simulink model "carModel"  (R2021a)
settings: Solver=ode15s  StartTime=0.0  StopTime=50  MaxStep=0.5  RelTol=1e-3
values from neighbouring files (symbols this model uses):
  initialFuel = 100    [data.m]
  maxEngineTemp = 240    [data.m]
  maxEngineTorque = 80    [data.m]
  maxMotorTemp = 135    [data.m]
  maxMotorTorque = 80    [data.m]
  maxRegenTorque = 80    [data.m]
  motorVoltage = 140    [data.m]
undefined symbols (not defined in the file or in its folder): b, k, Lock, N, sigbuilder_block, Temp_bpts, up
libraries: autolibsharedcoupling x7, autolibshared x7, autolibpowerinfoutils x4, autolibshareddiff x3, autolibhevctrlrcommon x2, autolibtrqconv x2, autolibutils x2, autolibtransamt x1, autolibsharedtransfixedgear x1, autolibdcdc x1, autolibdatasheetbattery x1, autolibmappedmotor x1
(part 6 of 6)

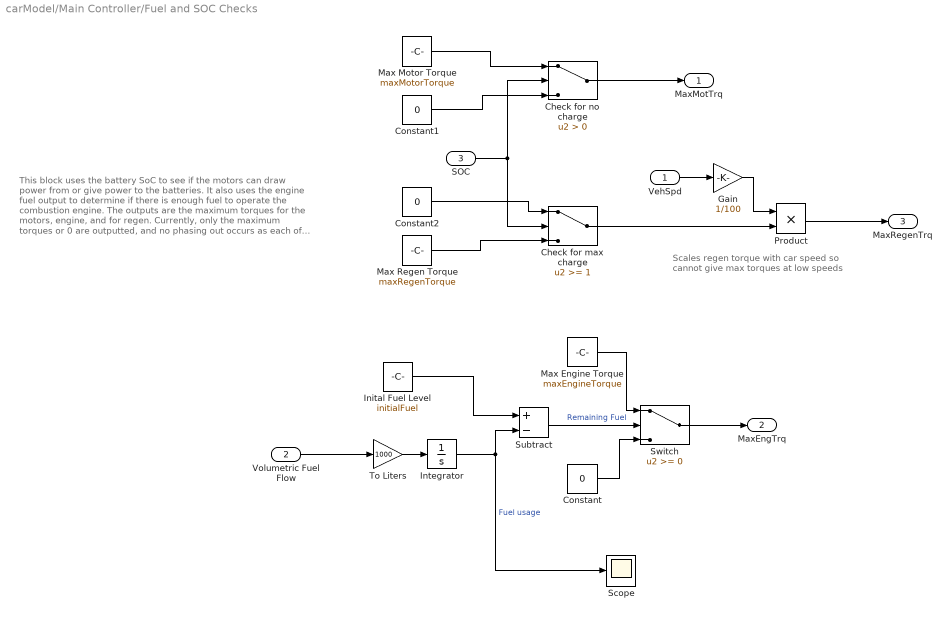
== system carModel/Main Controller/Fuel and SOC Checks ==
  note: Scales regen torque with car speed
      | so cannot give max torques at low speeds
  note: This block uses the battery SoC to see if the motors can draw power from or give power to the batteries. It also uses the engine fuel output to determine if there is enough fuel to operate the combustion engine. The outputs are the maximum torques for the motors, engine, and for regen.
      |
      | Currently, only the maximum torques or 0 are outputted, and no phasing out occurs as each of the power supply decreases.
  VehSpd : Inport
  Volumetric Fuel Flow : Inport  Port=2
  SOC : Inport  Port=3
  Check for max charge : Switch  Threshold=1
  Check for no charge : Switch  Criteria=u2 > Threshold
  Constant : Constant  Value=0
  Constant1 : Constant  Value=0
  Constant2 : Constant  Value=0
  Gain : Gain  Gain=1/100
  Inital Fuel Level : Constant  Value=initialFuel
  Integrator : Integrator
  Max Engine Torque : Constant  Value=maxEngineTorque
  Max Motor Torque : Constant  Value=maxMotorTorque
  Max Regen Torque : Constant  Value=maxRegenTorque
  Product : Product
  Scope : Scope
  Subtract : Sum  Inputs=+-
  Switch : Switch
  To Liters : Gain  Gain=1000
  MaxMotTrq : Outport
  MaxEngTrq : Outport  Port=2
  MaxRegenTrq : Outport  Port=3
  wires:
  Subtract/1 -> Switch/2  "Remaining Fuel"
  Constant/1 -> Switch/3
  Inital Fuel Level/1 -> Subtract/1
  Integrator/1 -> Scope/1, Subtract/2  "Fuel usage"
  Volumetric Fuel Flow/1 -> To Liters/1
  Max Engine Torque/1 -> Switch/1
  Switch/1 -> MaxEngTrq/1
  Check for no charge/1 -> MaxMotTrq/1
  Max Motor Torque/1 -> Check for no charge/1
  Constant1/1 -> Check for no charge/3
  SOC/1 -> Check for max charge/2, Check for no charge/2
  Max Regen Torque/1 -> Check for max charge/3
  Constant2/1 -> Check for max charge/1
  Check for max charge/1 -> Product/2
  VehSpd/1 -> Gain/1
  Product/1 -> MaxRegenTrq/1
  Gain/1 -> Product/1
  To Liters/1 -> Integrator/1

== system carModel/Main Controller/Heat Controller ==
  note: Decreases the torque to the motor or engine if they are overheating by the power of the stand-in gain function.
      | This system doesn't make the other motor/engine work harder if one is too hot. Therefore when one is overheated the car instantly loses power, instead of when both are overheated.
  Motor Torque : Inport
  Engine Torque : Inport  Port=2
  Engine Temp Switch : Switch  Criteria=u2 > Threshold  Threshold=maxEngineTemp
  Motor Temp Switch : Switch  Criteria=u2 > Threshold  Threshold=maxMotorTemp
  Signal Builder : Subsystem  Tag=STV Subsys  LoadFcn=sigbuilder_block('load');  StartFcn=sigbuilder_block('start');  StopFcn=sigbuilder_block('stop');  ClipboardFcn=sigbuilder_block('clipboard');  mask(Sigbuilder block){tuvar=[0:10]}
      mask help: Simulink:masks:SigbuilderBlock_MD
      mask init:
      | if ~strcmp(get_param(bdroot(gcbh),'SimulationStatus'),'stopped') tuvar = sigbuilder_block('maskInit'); end
      settings: CopyFcn=sigbuilder_block('copy');  DeleteFcn=sigbuilder_block('delete');  ModelCloseFcn=sigbuilder_block('modelClose');  PreSaveFcn=sigbuilder_block('preSave');  PauseFcn=sigbuilder_block('pause');  ContinueFcn=sigbuilder_block('continue');  NameChangeFcn=sigbuilder_block('namechange');  OpenFcn=sigbuilder_block('open',[411 128.5 543.5 351.5 ]);  CloseFcn=sigbuilder_block('close');
      mask Display: plot(0, 0, 100, 100,[2, 2, 32, 32, 2], [68, 8, 8, 68, 68],[32, 2], [38, 38], [32, 19, 2],[53, 60, 44], [32, 17, 17, 2],[16, 16, 31, 31]);txt = getActiveGroup(gcbh);text(2, 100, txt,'verticalAlignment', 'top');
  place-holder to decrease engine torque : Gain
  place-holder to decrease motor torque : Gain
  Updated Motor Torque : Outport
  Updated Engine Torque : Outport  Port=2
  wires:
  Motor Torque/1 -> place-holder to decrease motor torque/1, Motor Temp Switch/3
  place-holder to decrease motor torque/1 -> Motor Temp Switch/1
  Engine Torque/1 -> place-holder to decrease engine torque/1, Engine Temp Switch/3
  place-holder to decrease engine torque/1 -> Engine Temp Switch/1
  Signal Builder/1(Motor temp) -> Motor Temp Switch/2
  Signal Builder/2(Engine temp) -> Engine Temp Switch/2
  Motor Temp Switch/1 -> Updated Motor Torque/1
  Engine Temp Switch/1 -> Updated Engine Torque/1

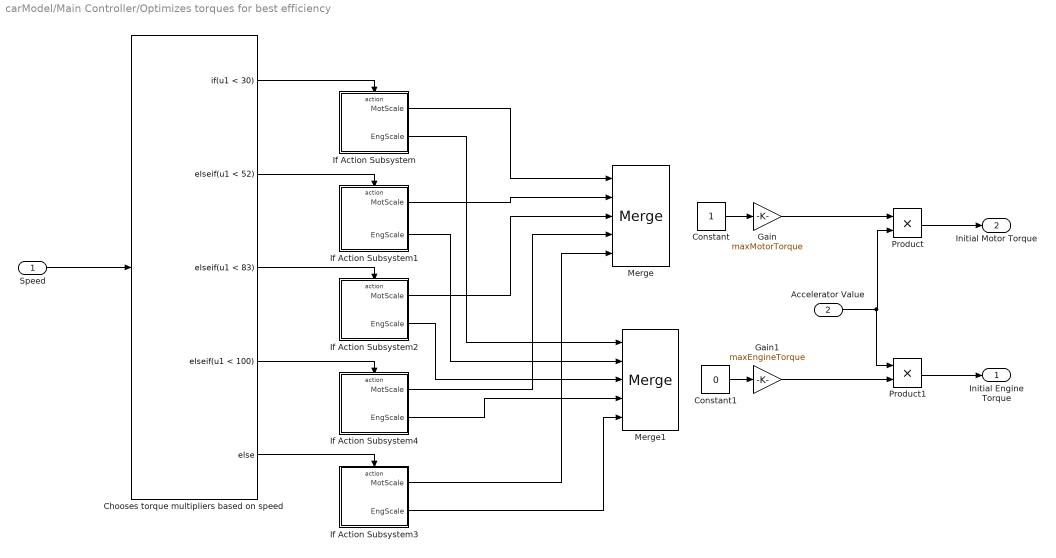
== system carModel/Main Controller/Optimizes torques for best efficiency ==
  Speed : Inport
  Accelerator Value : Inport  Port=2
  Chooses torque multipliers based on speed : If  IfExpression=u1 < 30  ElseIfExpressions=u1 < 52, u1 < 83, u1 < 100
  Constant : Constant
  Constant1 : Constant  Value=0
  Gain : Gain  Gain=maxMotorTorque
  Gain1 : Gain  Gain=maxEngineTorque
  If Action Subsystem : Subsystem  TreatAsAtomicUnit=on
  If Action Subsystem1 : Subsystem  TreatAsAtomicUnit=on
  If Action Subsystem2 : Subsystem  TreatAsAtomicUnit=on
  If Action Subsystem3 : Subsystem  TreatAsAtomicUnit=on
  If Action Subsystem4 : Subsystem  TreatAsAtomicUnit=on
  Merge : Merge  Inputs=5
  Merge1 : Merge  Inputs=5
  Product : Product
  Product1 : Product
  Initial Engine Torque : Outport
  Initial Motor Torque : Outport  Port=2
  wires:
  Speed/1 -> Chooses torque multipliers based on speed/1
  Accelerator Value/1 -> Product1/1, Product/2
  Product1/1 -> Initial Engine Torque/1
  Product/1 -> Initial Motor Torque/1
  Gain1/1 -> Product1/2
  Gain/1 -> Product/1
  Chooses torque multipliers based on speed/1 -> If Action Subsystem/Action
  Chooses torque multipliers based on speed/2 -> If Action Subsystem1/Action
  Chooses torque multipliers based on speed/3 -> If Action Subsystem2/Action
  Chooses torque multipliers based on speed/4 -> If Action Subsystem4/Action
  Chooses torque multipliers based on speed/5 -> If Action Subsystem3/Action
  If Action Subsystem/1(MotScale) -> Merge/1
  If Action Subsystem1/1(MotScale) -> Merge/2
  If Action Subsystem2/1(MotScale) -> Merge/3
  If Action Subsystem4/1(MotScale) -> Merge/4
  If Action Subsystem3/1(MotScale) -> Merge/5
  If Action Subsystem/2(EngScale) -> Merge1/1
  If Action Subsystem1/2(EngScale) -> Merge1/2
  If Action Subsystem2/2(EngScale) -> Merge1/3
  If Action Subsystem4/2(EngScale) -> Merge1/4
  If Action Subsystem3/2(EngScale) -> Merge1/5
  Constant/1 -> Gain/1
  Constant1/1 -> Gain1/1

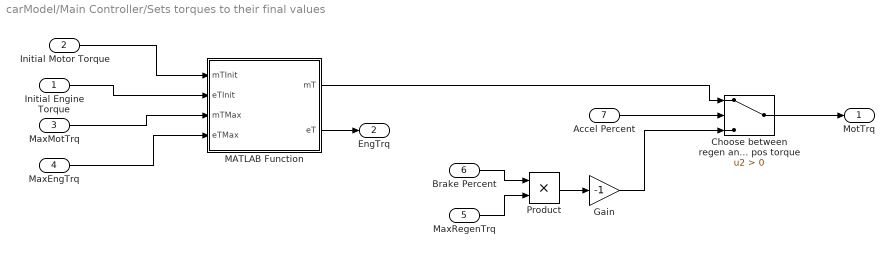
== system carModel/Main Controller/Sets torques to their final values ==
  Initial Engine Torque : Inport
  Initial Motor Torque : Inport  Port=2
  MaxMotTrq : Inport  Port=3
  MaxEngTrq : Inport  Port=4
  MaxRegenTrq : Inport  Port=5
  Brake Percent : Inport  Port=6
  Accel Percent : Inport  Port=7
  Choose between regen and pos torque : Switch  Criteria=u2 > Threshold
  Gain : Gain  Gain=-1
  MATLAB Function : MATLAB Function  TreatAsAtomicUnit=on
  Product : Product
  MotTrq : Outport
  EngTrq : Outport  Port=2
  wires:
  Gain/1 -> Choose between regen and pos torque/3
  MaxMotTrq/1 -> MATLAB Function/3(mTMax)
  MaxEngTrq/1 -> MATLAB Function/4(eTMax)
  Product/1 -> Gain/1
  Choose between regen and pos torque/1 -> MotTrq/1
  Brake Percent/1 -> Product/1
  Accel Percent/1 -> Choose between regen and pos torque/2
  MaxRegenTrq/1 -> Product/2
  Initial Motor Torque/1 -> MATLAB Function/1(mTInit)
  Initial Engine Torque/1 -> MATLAB Function/2(eTInit)
  MATLAB Function/2(eT) -> EngTrq/1
  MATLAB Function/1(mT) -> Choose between regen and pos torque/1

== system carModel/SI Engine/Accessory Load Model ==
  EngTrqIn : Inport
  EngSpd : Inport  Port=2
  Accessory Load Model : autolibhevctrlrcommon/Accessory Load Model  AccPwrTbl=[0 0]  AccSpdBpts=[300 750]
      settings: SourceProductBaseCode=PW
  Lumped Torque Dynamics : TransferFcn  Denominator=[0.2 1]
  Net Torque : Sum  Inputs=+-
  EngTrqOut : Outport  Unit=N*m  VectorParamsAs1DForOutWhenUnconnected=off
  wires:
  EngSpd/1 -> Accessory Load Model/1
  Lumped Torque Dynamics/1 -> EngTrqOut/1
  Net Torque/1 -> Lumped Torque Dynamics/1
  EngTrqIn/1 -> Net Torque/1
  Accessory Load Model/1 -> Net Torque/2

== system carModel/Drivetrain/Differential/Rear Axle Compliance 2 ==
  Info : Inport
  Bus Selector1 : BusSelector  OutputSignals=Trq.R,Trq.C
  Terminator : Terminator
  Terminator1 : Terminator
  Two-Way Connection1 : TwoWayConnection
  Two-Way Connection4 : TwoWayConnection
  R : PMIOPort  Side=Left
  C : PMIOPort  Port=2  Side=Right
  wires:
  Bus Selector1/2 -> Two-Way Connection1/1  "<C>"
  Bus Selector1/1 -> Two-Way Connection4/1  "<R>"
  Two-Way Connection1/1 -> Terminator1/1
  Info/1 -> Bus Selector1/1
  Two-Way Connection4/1 -> Terminator/1
  connections:
  Two-Way Connection1/RConn1 -- C/RConn1
  R/RConn1 -- Two-Way Connection4/RConn1

== system carModel/Drivetrain/Differential and Compliance/Front Axle Compliance 2 ==
  Info : Inport
  Bus Selector : BusSelector  OutputSignals=PwrInfo.PwrTrnsfrd,PwrInfo.PwrNotTrnsfrd,PwrInfo.PwrStored
  Bus Selector1 : BusSelector  OutputSignals=Trq.R,Trq.C
  Power Accounting Bus Creator : autolibpowerinfoutils/Power Accounting Bus Creator  AssctBlkSelPopup=Parent  RefBlkName='libraryname/blkname'  PwrTrnsfrdCheckBox=on  PwrNotTrnsfrdCheckBox=on  PwrStoredCheckBox=on  aMode=aMode
      settings: SourceProductBaseCode=PW,DR,MT,UV,VE
  Terminator : Terminator
  Terminator1 : Terminator
  Terminator2 : Terminator
  Two-Way Connection1 : TwoWayConnection
  Two-Way Connection4 : TwoWayConnection
  R : PMIOPort  Side=Left
  C : PMIOPort  Port=2  Side=Right
  wires:
  Bus Selector/3 -> Power Accounting Bus Creator/3  "<PwrStored>"
  Bus Selector/2 -> Power Accounting Bus Creator/2  "<PwrNotTrnsfrd>"
  Bus Selector/1 -> Power Accounting Bus Creator/1  "<PwrTrnsfrd>"
  Power Accounting Bus Creator/1 -> Terminator2/1
  Bus Selector1/2 -> Two-Way Connection1/1  "<C>"
  Bus Selector1/1 -> Two-Way Connection4/1  "<R>"
  Two-Way Connection1/1 -> Terminator1/1
  Info/1 -> Bus Selector/1, Bus Selector1/1
  Two-Way Connection4/1 -> Terminator/1
  connections:
  Two-Way Connection1/RConn1 -- C/RConn1
  R/RConn1 -- Two-Way Connection4/RConn1

== system carModel/Drivetrain/Differential and Compliance/Rear Axle Compliance 2 ==
  Info : Inport
  Bus Selector : BusSelector  OutputSignals=PwrInfo.PwrTrnsfrd,PwrInfo.PwrNotTrnsfrd,PwrInfo.PwrStored
  Bus Selector1 : BusSelector  OutputSignals=Trq.R,Trq.C
  Power Accounting Bus Creator : autolibpowerinfoutils/Power Accounting Bus Creator  AssctBlkSelPopup=Parent  RefBlkName='libraryname/blkname'  PwrTrnsfrdCheckBox=on  PwrNotTrnsfrdCheckBox=on  PwrStoredCheckBox=on  aMode=aMode
      settings: SourceProductBaseCode=PW,DR,MT,UV,VE
  Terminator : Terminator
  Terminator1 : Terminator
  Terminator2 : Terminator
  Two-Way Connection1 : TwoWayConnection
  Two-Way Connection4 : TwoWayConnection
  R : PMIOPort  Side=Left
  C : PMIOPort  Port=2  Side=Right
  wires:
  Bus Selector/3 -> Power Accounting Bus Creator/3  "<PwrStored>"
  Bus Selector/2 -> Power Accounting Bus Creator/2  "<PwrNotTrnsfrd>"
  Bus Selector/1 -> Power Accounting Bus Creator/1  "<PwrTrnsfrd>"
  Power Accounting Bus Creator/1 -> Terminator2/1
  Bus Selector1/2 -> Two-Way Connection1/1  "<C>"
  Bus Selector1/1 -> Two-Way Connection4/1  "<R>"
  Two-Way Connection1/1 -> Terminator1/1
  Info/1 -> Bus Selector/1, Bus Selector1/1
  Two-Way Connection4/1 -> Terminator/1
  connections:
  Two-Way Connection1/RConn1 -- C/RConn1
  R/RConn1 -- Two-Way Connection4/RConn1

== system carModel/Drivetrain/Transmission/Accessory Load Model1 ==
  EngTrqIn : Inport
  EngSpd : Inport  Port=2
  Accessory Load Model : autolibhevctrlrcommon/Accessory Load Model  AccPwrTbl=[0 0]  AccSpdBpts=[300 750]
      settings: SourceProductBaseCode=PW
  Lumped Torque Dynamics : TransferFcn  Denominator=[0.2 1]
  Net Torque : Sum  Inputs=+-
  EngTrqOut : Outport  Unit=N*m  VectorParamsAs1DForOutWhenUnconnected=off
  wires:
  EngSpd/1 -> Accessory Load Model/1
  Lumped Torque Dynamics/1 -> EngTrqOut/1
  Net Torque/1 -> Lumped Torque Dynamics/1
  EngTrqIn/1 -> Net Torque/1
  Accessory Load Model/1 -> Net Torque/2

== system carModel/Drivetrain/Transmission/Subsystem ==
  note: Gear Selection based on current vehicle speed
  VehSpdFdbk : Inport
  Gear 0 : Subsystem  TreatAsAtomicUnit=on
  Gear 1 : Subsystem  TreatAsAtomicUnit=on
  Gear 2 : Subsystem  TreatAsAtomicUnit=on
  Gear 3 : Subsystem  TreatAsAtomicUnit=on
  Gear 4 : Subsystem  TreatAsAtomicUnit=on
  Gear 5 : Subsystem  TreatAsAtomicUnit=on
  Gear Chooser : If  IfExpression=u1 == 0  ElseIfExpressions=u1 < 49.31, u1 < 60.69, u1 < 73.70, u1 < 88.70
  Selected Gear Merger : Merge  Inputs=6
  Gear : Outport
  wires:
  VehSpdFdbk/1 -> Gear Chooser/1
  Selected Gear Merger/1 -> Gear/1
  Gear 1/1(Out1) -> Selected Gear Merger/2
  Gear 2/1(Out1) -> Selected Gear Merger/3
  Gear 3/1(Out1) -> Selected Gear Merger/4
  Gear 4/1(Out1) -> Selected Gear Merger/5
  Gear 5/1(Out1) -> Selected Gear Merger/6
  Gear Chooser/5 -> Gear 4/Action
  Gear Chooser/6 -> Gear 5/Action
  Gear Chooser/4 -> Gear 3/Action
  Gear Chooser/3 -> Gear 2/Action
  Gear Chooser/2 -> Gear 1/Action
  Gear Chooser/1 -> Gear 0/Action
  Gear 0/1(Out1) -> Selected Gear Merger/1

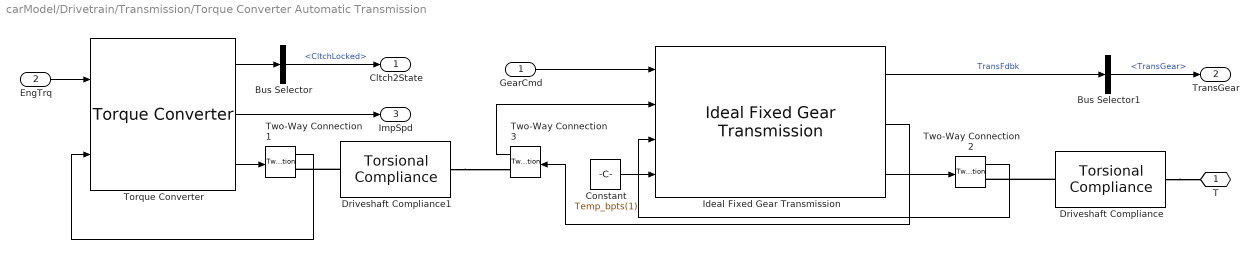
== system carModel/Drivetrain/Transmission/Torque Converter Automatic Transmission ==
  GearCmd : Inport
  EngTrq : Inport  Port=2
  Bus Selector : BusSelector  OutputSignals=Cltch.CltchLocked
  Bus Selector1 : BusSelector  OutputSignals=Trans.TransGear
  Constant : Constant  Value=Temp_bpts(1)
  Driveshaft Compliance : autolibsharedcoupling/Torsional Compliance  port_config=Two-way connection  extInfo=off  k=k  b=b  theta_o=theta_o  domega_o=domega_o  omega_c=omega_c  blkID=0  aMode=1
      settings: SourceProductBaseCode=PW,DR,MT,UV,VE
  Driveshaft Compliance1 : autolibsharedcoupling/Torsional Compliance  port_config=Two-way connection  extInfo=off  k=k  b=b  theta_o=theta_o  domega_o=domega_o  omega_c=omega_c  blkID=0  aMode=1
      settings: SourceProductBaseCode=PW,DR,MT,UV,VE
  Ideal Fixed Gear Transmission : autolibsharedtransfixedgear/Ideal Fixed Gear Transmission  VariantControl=0  TransEffModelPopup=Gear, input torque, input speed, and temperature  gearInterp=Linear point-slope  G=G  Trq_bpts=Trq_bpts  omega_bpts=omega_bpts  Temp_bpts=Temp_bpts  N=N  Jout=Jout  bout=bout  eta=eta  eta_tbl=eta_tbl  G_o=0  omega_o=omega_o  omegaN_o=0  tau_s=tau_s  maxAbsSpd=5e3  aMode=1
      settings: SourceProductBaseCode=PW,DR,MT,UV,VE
  Torque Converter : autolibtrqconv/Torque Converter  TCType=Lock-up  port_config=Simulink  Ji=Ji  bi=bi  Jt=Jt  bt=bt  omegai_o=omegai_o  omegat_o=omegat_o  phi=phi  KType=Input speed / sqrt(input torque)  psi=psi  zeta=zeta  tauTC=tauTC  InterpMethod=Linear  Reff=Reff  mus=mus  muk=muk  ClutchLocked=off  philu=philu  omegal=omegal  omegau=omegau  K_c=K_c  tauC=tauC  maxAbsSpd=5e3  tau_dl=3000
      settings: AttributesFormatString="Lock-up type:  %<TCType>"  SourceProductBaseCode=PW
  Two-Way Connection1 : TwoWayConnection
  Two-Way Connection2 : TwoWayConnection
  Two-Way Connection3 : TwoWayConnection
  T : PMIOPort  Side=Right
  Cltch2State : Outport  VectorParamsAs1DForOutWhenUnconnected=off
  TransGear : Outport  Port=2  VectorParamsAs1DForOutWhenUnconnected=off
  ImpSpd : Outport  Port=3  VectorParamsAs1DForOutWhenUnconnected=off
  wires:
  Bus Selector1/1 -> TransGear/1  "<TransGear>"
  Constant/1 -> Ideal Fixed Gear Transmission/4
  Bus Selector/1 -> Cltch2State/1  "<CltchLocked>"
  Two-Way Connection3/1 -> Ideal Fixed Gear Transmission/2
  EngTrq/1 -> Torque Converter/1
  Ideal Fixed Gear Transmission/3 -> Two-Way Connection2/1
  Two-Way Connection1/1 -> Torque Converter/2
  Two-Way Connection2/1 -> Ideal Fixed Gear Transmission/3
  Torque Converter/3 -> Two-Way Connection1/1
  Ideal Fixed Gear Transmission/2 -> Two-Way Connection3/1
  Torque Converter/1 -> Bus Selector/1
  Torque Converter/2 -> ImpSpd/1
  Ideal Fixed Gear Transmission/1 -> Bus Selector1/1  "TransFdbk"
  GearCmd/1 -> Ideal Fixed Gear Transmission/1
  connections:
  Driveshaft Compliance/RConn1 -- T/RConn1
  Driveshaft Compliance1/LConn1 -- Two-Way Connection1/RConn1
  Driveshaft Compliance/LConn1 -- Two-Way Connection2/RConn1
  Driveshaft Compliance1/RConn1 -- Two-Way Connection3/RConn1

== system carModel/Drivetrain/Wheels and Brakes2/Longitudinal Wheel - Front 2 ==
  Info : Inport
  AxlTrq : Inport  Port=2
  Vx : Inport  Port=3
  Fz : Inport  Port=4
  Bus Selector : BusSelector  OutputSignals=PwrInfo.PwrTrnsfrd,PwrInfo.PwrNotTrnsfrd,PwrInfo.PwrStored,Fx,Omega
  Power Accounting Bus Creator : autolibpowerinfoutils/Power Accounting Bus Creator  AssctBlkSelPopup=Parent  RefBlkName='libraryname/blkname'  PwrTrnsfrdCheckBox=on  PwrNotTrnsfrdCheckBox=on  PwrStoredCheckBox=on  aMode=aMode
      settings: SourceProductBaseCode=PW,DR,MT,UV,VE
  Terminator{,1..3} (4 alike) : Terminator
  Fx : Outport  VectorParamsAs1DForOutWhenUnconnected=off
  Omega : Outport  Port=2  VectorParamsAs1DForOutWhenUnconnected=off
  wires:
  Power Accounting Bus Creator/1 -> Terminator3/1
  Bus Selector/5 -> Omega/1  "<Omega>"
  Bus Selector/4 -> Fx/1  "<Fx>"
  Bus Selector/3 -> Power Accounting Bus Creator/3  "<PwrStored>"
  Bus Selector/2 -> Power Accounting Bus Creator/2  "<PwrNotTrnsfrd>"
  Bus Selector/1 -> Power Accounting Bus Creator/1  "<PwrTrnsfrd>"
  Info/1 -> Bus Selector/1
  Fz/1 -> Terminator2/1
  Vx/1 -> Terminator1/1
  AxlTrq/1 -> Terminator/1

== system carModel/Drivetrain/Wheels and Brakes2/Longitudinal Wheel - Rear 2 ==
  Info : Inport
  AxlTrq : Inport  Port=2
  Vx : Inport  Port=3
  Fz : Inport  Port=4
  Bus Selector : BusSelector  OutputSignals=PwrInfo.PwrTrnsfrd,PwrInfo.PwrNotTrnsfrd,PwrInfo.PwrStored,Fx,Omega
  Power Accounting Bus Creator : autolibpowerinfoutils/Power Accounting Bus Creator  AssctBlkSelPopup=Parent  RefBlkName='libraryname/blkname'  PwrTrnsfrdCheckBox=on  PwrNotTrnsfrdCheckBox=on  PwrStoredCheckBox=on  aMode=aMode
      settings: SourceProductBaseCode=PW,DR,MT,UV,VE
  Terminator{,1..3} (4 alike) : Terminator
  Fx : Outport  VectorParamsAs1DForOutWhenUnconnected=off
  Omega : Outport  Port=2  VectorParamsAs1DForOutWhenUnconnected=off
  wires:
  Power Accounting Bus Creator/1 -> Terminator3/1
  Bus Selector/5 -> Omega/1  "<Omega>"
  Bus Selector/4 -> Fx/1  "<Fx>"
  Bus Selector/3 -> Power Accounting Bus Creator/3  "<PwrStored>"
  Bus Selector/2 -> Power Accounting Bus Creator/2  "<PwrNotTrnsfrd>"
  Bus Selector/1 -> Power Accounting Bus Creator/1  "<PwrTrnsfrd>"
  Info/1 -> Bus Selector/1
  Fz/1 -> Terminator2/1
  Vx/1 -> Terminator1/1
  AxlTrq/1 -> Terminator/1

== system carModel/Main Controller/Heat Controller/Signal Builder ==
  Demux : Demux  Tag=STV Demux  Outputs=2
      settings: DisplayOption=none
  FromWs : FromWorkspace  Tag=STV FromWs  VariableName=tuvar
      SigBuilderData=|
      | common.afterFinalStr = 'Extrapolate'
      | common.sampleTime = 0
      | dataSet.timeRange = [0 10]
      | dataSet.name = 'Temperature Signals'
      | sbobj.Groups.Name = 'Temperature Signals'
      | sbobj.Groups.Signals(1).Name = 'Motor temp'
      | sbobj.Groups.Signals(1).XData = [0 10]
      | sbobj.Groups.Signals(1).YData = [0 0]
      | sbobj.Groups.Signals(2).Name = 'Engine temp'
      | sbobj.Groups.Signals(2).XData = [0 10]
      | sbobj.Groups.Signals(2).YData = [0 0]
  Motor temp : Outport  Tag=STV Outport
  Engine temp : Outport  Tag=STV Outport  Port=2
  wires:
  FromWs/1 -> Demux/1
  Demux/1 -> Motor temp/1
  Demux/2 -> Engine temp/1

== system carModel/Main Controller/Optimizes torques for best efficiency/If Action Subsystem ==
  Action Port : ActionPort  ActionPortLabel=if(u1 < 30)
  Constant : Constant  Value=0
  Constant1 : Constant
  MotScale : Outport
  EngScale : Outport  Port=2
  wires:
  Constant/1 -> MotScale/1
  Constant1/1 -> EngScale/1

== system carModel/Main Controller/Optimizes torques for best efficiency/If Action Subsystem1 ==
  Action Port : ActionPort  ActionPortLabel=elseif(u1 < 52)
  Constant : Constant  Value=0
  Constant1 : Constant
  MotScale : Outport
  EngScale : Outport  Port=2
  wires:
  Constant/1 -> MotScale/1
  Constant1/1 -> EngScale/1

== system carModel/Main Controller/Optimizes torques for best efficiency/If Action Subsystem2 ==
  Action Port : ActionPort  ActionPortLabel=elseif( u1 < 83)
  Constant : Constant  Value=0
  Constant1 : Constant
  MotScale : Outport
  EngScale : Outport  Port=2
  wires:
  Constant1/1 -> EngScale/1
  Constant/1 -> MotScale/1

== system carModel/Main Controller/Optimizes torques for best efficiency/If Action Subsystem3 ==
  Action Port : ActionPort  ActionPortLabel=else
  Constant : Constant  Value=0
  Constant1 : Constant  Value=0
  MotScale : Outport
  EngScale : Outport  Port=2
  wires:
  Constant1/1 -> EngScale/1
  Constant/1 -> MotScale/1

== system carModel/Main Controller/Optimizes torques for best efficiency/If Action Subsystem4 ==
  Action Port : ActionPort  ActionPortLabel=elseif( u1 < 100)
  Constant : Constant  Value=0
  Constant1 : Constant
  MotScale : Outport
  EngScale : Outport  Port=2
  wires:
  Constant1/1 -> EngScale/1
  Constant/1 -> MotScale/1

== system carModel/Drivetrain/Transmission/Subsystem/Gear 0 ==
  Action Port : ActionPort  ActionPortLabel=if(u1 == 0)
  Constant : Constant  Value=0
  Out1 : Outport
  wires:
  Constant/1 -> Out1/1

== system carModel/Drivetrain/Transmission/Subsystem/Gear 1 ==
  Action Port : ActionPort  ActionPortLabel=elseif(u1 < 49.31)
  Constant : Constant
  Out1 : Outport
  wires:
  Constant/1 -> Out1/1

== system carModel/Drivetrain/Transmission/Subsystem/Gear 2 ==
  Action Port : ActionPort  ActionPortLabel=elseif( u1 < 60.69)
  Constant : Constant  Value=2
  Out1 : Outport
  wires:
  Constant/1 -> Out1/1

== system carModel/Drivetrain/Transmission/Subsystem/Gear 3 ==
  Action Port : ActionPort  ActionPortLabel=elseif( u1 < 73.70)
  Constant : Constant  Value=3
  Out1 : Outport
  wires:
  Constant/1 -> Out1/1

== system carModel/Drivetrain/Transmission/Subsystem/Gear 4 ==
  Action Port : ActionPort  ActionPortLabel=elseif( u1 < 88.70)
  Constant : Constant  Value=4
  Out1 : Outport
  wires:
  Constant/1 -> Out1/1

== system carModel/Drivetrain/Transmission/Subsystem/Gear 5 ==
  Action Port : ActionPort  ActionPortLabel=else
  Constant : Constant  Value=5
  Out1 : Outport
  wires:
  Constant/1 -> Out1/1

== matlab function carModel/Main Controller/Sets torques to their final values/MATLAB Function ==
  data: mTInit input; mT output; eTInit input; mTMax input; eTMax input; eT output
function [mT, eT] = fcn(mTInit, eTInit, mTMax, eTMax)
if (mTInit <= mTMax && eTInit <= eTMax) % both initial supplies are valid
    mT = mTInit;
    eT = eTInit;
elseif (mTInit > mTMax && eTInit <= eTMax) % motor torque is too high
    mT = mTMax;
    engSpace = (eTMax - eTInit);
    motOver = (mTInit - mTMax);
    if (engSpace > motOver) 
        eT = eTInit + motOver;
    else
        eT = eTMax;
    end
elseif (mTInit <= mTMax && eTInit > eTMax) % engine torue is too high
    eT = eTMax;
    motSpace = (mTMax - mTInit);
    engOver = (eTInit - eTMax);
    if (motSpace > engOver) 
        mT = mTInit + engOver;
    else
        mT = mTMax;
    end
else % both torques are too high
    mT = mTMax;
    eT = eTMax;
end
end
